simulink model "sim_SoftwareIntheLoop_Compensator"  (R2018a)
settings: Solver=ode3  StartTime=0.0  StopTime=40  FixedStep=0.005  RelTol=1e-3  EnableMultiTasking=on
InitFcn:
  | % load parameters of the default quadrotor
  | disp('Quadrotor parameters loaded by InitFcn')
  | parameters_estimationcontrol %load mdl_quadcopter as well!
  | 
  | % change to Simulation folder if in data folder
  | %cd([matlabpath '/Simulation']);
values from neighbouring files (symbols this model uses):
  controlHelperParams =     [LQR_param.mat]
  estimParams =     [LQR_param.mat]
  quad =     [LQR_param.mat]
  quadEDT =     [LQR_param.mat]
undefined symbols (not defined in the file or in its folder): DiscIntNeverNeededParam, Discrete, RSrun_sensordataCalib, rt_yout, Time
libraries: simulink x25, ctrlSharedLib x3
(part 1 of 2)
settings Model: Creator=ra  LastModifiedBy=Tony
settings DataIOCC: LimitDataPoints=on  SaveFormat=Array
settings OptimizationCC: LifeSpan=inf
settings DebuggingCC: SFUnexpectedBacktrackingDiag=warning  SFNoUnconditionalDefaultTransitionDiag=warning  SFExecutionAtInitializationDiag=none
settings HardwareCC: ProdBitPerPointer=32  ProdBitPerSizeT=32  ProdBitPerPtrDiffT=32  ProdLargestAtomicFloat=None  ProdIntDivRoundTo=Undefined  ProdEndianess=Unspecified  ProdWordSize=32  ProdHWDeviceType=32-bit Generic
settings ModelReferenceCC: PropagateSignalLabelsOutOfModel=off
settings CodeAppCC: StateflowObjectComments=on
settings GRTTargetCC: TargetLangStandard=C89/C90 (ANSI)  GeneratePreprocessorConditionals=Disable all
settings ConfigComp: CovMetricSettings=dw  CovHtmlReporting=on  CovSaveCumulativeToWorkspaceVar=on  CovSaveSingleToWorkspaceVar=on  CovExternalEMLEnable=off

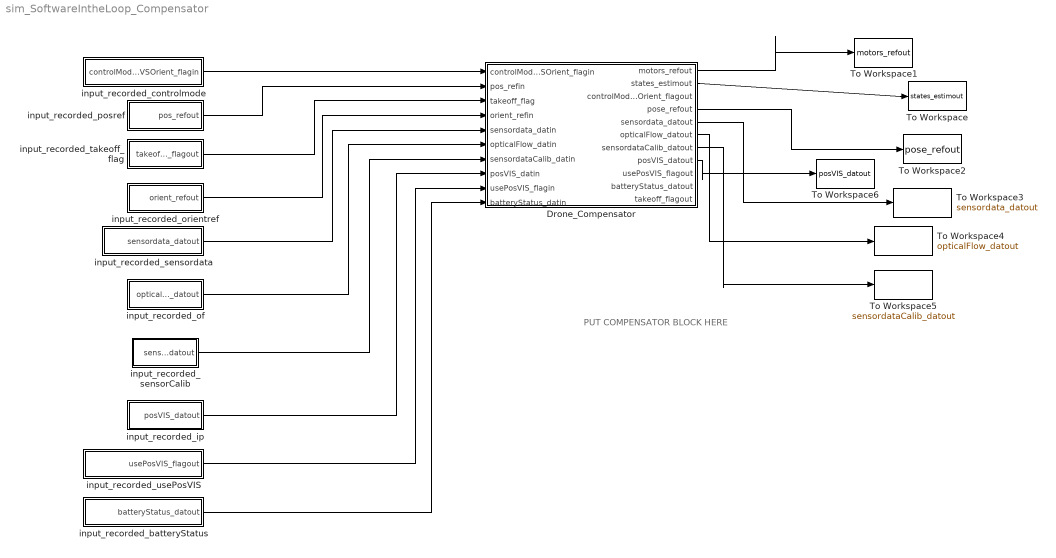
== system sim_SoftwareIntheLoop_Compensator ==
  note: PUT COMPENSATOR BLOCK HERE
  Drone_Compensator : Subsystem  TreatAsAtomicUnit=on
  To Workspace : ToWorkspace  VariableName=states_estimout  SaveFormat=Timeseries  SampleTime=-1
  To Workspace1 : ToWorkspace  VariableName=motors_refout  SaveFormat=Timeseries  SampleTime=-1
  To Workspace2 : ToWorkspace  VariableName=pose_refout  SaveFormat=Timeseries  SampleTime=-1
  To Workspace3 : ToWorkspace  VariableName=sensordata_datout  SaveFormat=Timeseries  SampleTime=-1
  To Workspace4 : ToWorkspace  VariableName=opticalFlow_datout  SaveFormat=Timeseries  SampleTime=-1
  To Workspace5 : ToWorkspace  VariableName=sensordataCalib_datout  SaveFormat=Timeseries  SampleTime=-1
  To Workspace6 : ToWorkspace  VariableName=posVIS_datout  SaveFormat=Timeseries  SampleTime=-1
  input_recorded_batteryStatus : Subsystem
  input_recorded_controlmode : Subsystem
  input_recorded_ip : Subsystem
  input_recorded_of : Subsystem
  input_recorded_orientref : Subsystem
  input_recorded_posref : Subsystem
  input_recorded_sensorCalib : Subsystem
  input_recorded_sensordata : Subsystem
  input_recorded_takeoff_flag : Subsystem
  input_recorded_usePosVIS : Subsystem
  wires:
  input_recorded_of/1(opticalFlow_datout) -> Drone_Compensator/6(opticalFlow_datin)
  input_recorded_sensordata/1(sensordata_datout) -> Drone_Compensator/5(sensordata_datin)
  input_recorded_ip/1(posVIS_datout) -> Drone_Compensator/8(posVIS_datin)
  input_recorded_orientref/1(orient_refout) -> Drone_Compensator/4(orient_refin)
  input_recorded_posref/1(pos_refout) -> Drone_Compensator/2(pos_refin)
  input_recorded_controlmode/1(controlModePosVSOrient_flagin) -> Drone_Compensator/1(controlModePosVSOrient_flagin)
  input_recorded_usePosVIS/1(usePosVIS_flagout) -> Drone_Compensator/9(usePosVIS_flagin)
  input_recorded_batteryStatus/1(batteryStatus_datout) -> Drone_Compensator/10(batteryStatus_datin)
  input_recorded_sensorCalib/1(sensordataCalib_datout) -> Drone_Compensator/7(sensordataCalib_datin)
  input_recorded_takeoff_flag/1(takeoff_flagout) -> Drone_Compensator/3(takeoff_flag)
  Drone_Compensator/2(states_estimout) -> To Workspace/1
  Drone_Compensator/1(motors_refout) -> To Workspace1/1
  Drone_Compensator/4(pose_refout) -> To Workspace2/1
  Drone_Compensator/5(sensordata_datout) -> To Workspace3/1
  Drone_Compensator/6(opticalFlow_datout) -> To Workspace4/1
  Drone_Compensator/7(sensordataCalib_datout) -> To Workspace5/1
  Drone_Compensator/8(posVIS_datout) -> To Workspace6/1

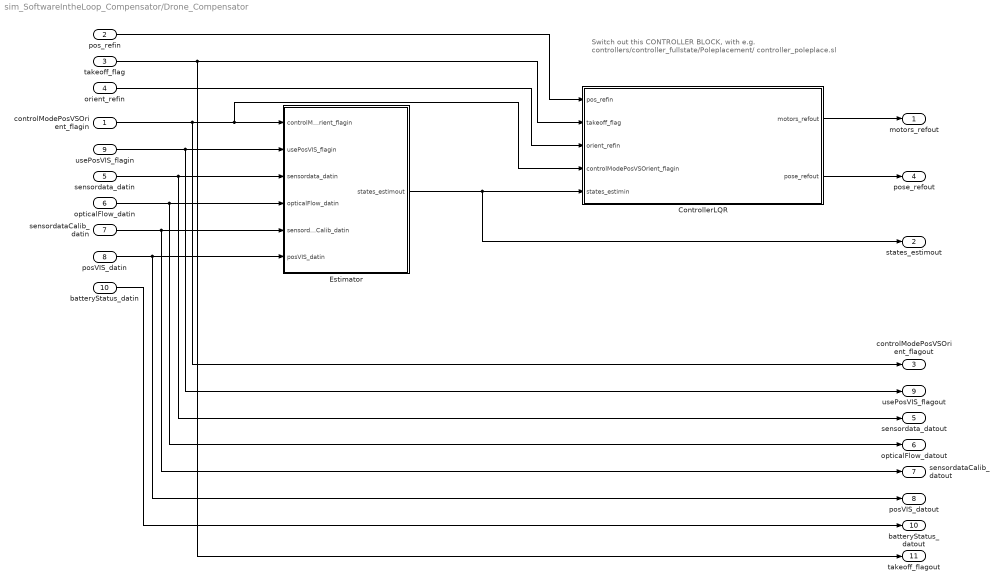
== system sim_SoftwareIntheLoop_Compensator/Drone_Compensator ==
  note: Switch out this CONTROLLER BLOCK, with e.g.
      | controllers/controller_fullstate/Poleplacement/
      | controller_poleplace.sl
  controlModePosVSOrient_flagin : Inport
  pos_refin : Inport  Port=2
  takeoff_flag : Inport  Port=3
  orient_refin : Inport  Port=4
  sensordata_datin : Inport  Port=5
  opticalFlow_datin : Inport  Port=6
  sensordataCalib_datin : Inport  Port=7
  posVIS_datin : Inport  Port=8
  usePosVIS_flagin : Inport  Port=9
  batteryStatus_datin : Inport  Port=10
  ControllerLQR : Subsystem  TreatAsAtomicUnit=on
  Estimator : Subsystem
  motors_refout : Outport
  states_estimout : Outport  Port=2
  controlModePosVSOrient_flagout : Outport  Port=3
  pose_refout : Outport  Port=4
  sensordata_datout : Outport  Port=5
  opticalFlow_datout : Outport  Port=6
  sensordataCalib_datout : Outport  Port=7
  posVIS_datout : Outport  Port=8
  usePosVIS_flagout : Outport  Port=9
  batteryStatus_datout : Outport  Port=10
  takeoff_flagout : Outport  Port=11
  wires:
  sensordata_datin/1 -> sensordata_datout/1, Estimator/3(sensordata_datin)
  pos_refin/1 -> ControllerLQR/1(pos_refin)
  Estimator/1(states_estimout) -> ControllerLQR/5(states_estimin), states_estimout/1
  orient_refin/1 -> ControllerLQR/3(orient_refin)
  controlModePosVSOrient_flagin/1 -> controlModePosVSOrient_flagout/1, ControllerLQR/4(controlModePosVSOrient_flagin), Estimator/1(controlModePosVSOrient_flagin)
  sensordataCalib_datin/1 -> sensordataCalib_datout/1, Estimator/5(sensordataCalib_datin)
  opticalFlow_datin/1 -> opticalFlow_datout/1, Estimator/4(opticalFlow_datin)
  posVIS_datin/1 -> posVIS_datout/1, Estimator/6(posVIS_datin)
  ControllerLQR/1(motors_refout) -> motors_refout/1
  usePosVIS_flagin/1 -> usePosVIS_flagout/1, Estimator/2(usePosVIS_flagin)
  ControllerLQR/2(pose_refout) -> pose_refout/1
  batteryStatus_datin/1 -> batteryStatus_datout/1
  takeoff_flag/1 -> ControllerLQR/2(takeoff_flag), takeoff_flagout/1

== system sim_SoftwareIntheLoop_Compensator/input_recorded_batteryStatus ==
  From Workspace : FromWorkspace  VariableName=RSrun_usePosVIS  SampleTime=quadEDT.sampletime
  Rate Transition : RateTransition  OutPortSampleTime=quadEDT.sampletime
  batteryStatus_datout : Outport
  wires:
  Rate Transition/1 -> batteryStatus_datout/1
  From Workspace/1 -> Rate Transition/1

== system sim_SoftwareIntheLoop_Compensator/input_recorded_controlmode ==
  From Workspace : FromWorkspace  VariableName=RSrun_controlMode  SampleTime=quadEDT.sampletime
  Rate Transition : RateTransition  OutPortSampleTime=quadEDT.sampletime
  controlModePosVSOrient_flagin : Outport
  wires:
  From Workspace/1 -> Rate Transition/1
  Rate Transition/1 -> controlModePosVSOrient_flagin/1

== system sim_SoftwareIntheLoop_Compensator/input_recorded_ip ==
  From Workspace : FromWorkspace  VariableName=RSrun_posVIS  SampleTime=quadEDT.sampletime
  Rate Transition : RateTransition  OutPortSampleTime=quadEDT.sampletime
  posVIS_datout : Outport
  wires:
  Rate Transition/1 -> posVIS_datout/1
  From Workspace/1 -> Rate Transition/1

== system sim_SoftwareIntheLoop_Compensator/input_recorded_of ==
  From Workspace : FromWorkspace  VariableName=RSrun_opticalFlow  SampleTime=quadEDT.sampletime
  Rate Transition : RateTransition  OutPortSampleTime=quadEDT.sampletime
  opticalFlow_datout : Outport
  wires:
  Rate Transition/1 -> opticalFlow_datout/1
  From Workspace/1 -> Rate Transition/1

== system sim_SoftwareIntheLoop_Compensator/input_recorded_orientref ==
  From Workspace : FromWorkspace  VariableName=RSrun_orient_ref  SampleTime=quadEDT.sampletime
  Rate Transition : RateTransition  OutPortSampleTime=quadEDT.sampletime
  orient_refout : Outport
  wires:
  From Workspace/1 -> Rate Transition/1
  Rate Transition/1 -> orient_refout/1

== system sim_SoftwareIntheLoop_Compensator/input_recorded_posref ==
  From Workspace : FromWorkspace  VariableName=RSrun_pos_ref  SampleTime=quadEDT.sampletime
  Rate Transition : RateTransition  OutPortSampleTime=quadEDT.sampletime
  pos_refout : Outport
  wires:
  Rate Transition/1 -> pos_refout/1
  From Workspace/1 -> Rate Transition/1

== system sim_SoftwareIntheLoop_Compensator/input_recorded_sensorCalib ==
  From Workspace : Constant  Value=RSrun_sensordataCalib  SampleTime=quadEDT.sampletime
  Rate Transition4 : RateTransition  OutPortSampleTime=quadEDT.sampletime
  sensorbias_default : Constant  Value=[0.09 -0.06 +0.337 -0.0095 -0.0075 0.0015 mean(rt_yout.signals(9).values(1:200))]  SampleTime=quadEDT.sampletime
  sensordataCalib_datout : Outport
  wires:
  From Workspace/1 -> Rate Transition4/1
  Rate Transition4/1 -> sensordataCalib_datout/1

== system sim_SoftwareIntheLoop_Compensator/input_recorded_sensordata ==
  Bus Creator : BusCreator  Inputs=8
  Demux : Demux  Outputs=8
  From Workspace : FromWorkspace  VariableName=RSrun_sensordata  SampleTime=quadEDT.sampletime
  Rate Transition : RateTransition  OutPortSampleTime=quadEDT.sampletime
  sensordata_datout : Outport
  wires:
  Demux/3 -> Bus Creator/3  "ddz"
  Demux/6 -> Bus Creator/6  "r"
  Demux/4 -> Bus Creator/4  "p"
  Demux/1 -> Bus Creator/1  "ddx"
  Demux/2 -> Bus Creator/2  "ddy"
  Bus Creator/1 -> Rate Transition/1
  Demux/5 -> Bus Creator/5  "q"
  From Workspace/1 -> Demux/1
  Demux/7 -> Bus Creator/7  "altitude_sonar"
  Rate Transition/1 -> sensordata_datout/1
  Demux/8 -> Bus Creator/8  "prs"

== system sim_SoftwareIntheLoop_Compensator/input_recorded_takeoff_flag ==
  From Workspace : FromWorkspace  VariableName=RSrun_takeoff_flag  SampleTime=quadEDT.sampletime
  Rate Transition : RateTransition  OutPortSampleTime=quadEDT.sampletime
  takeoff_flagout : Outport
  wires:
  Rate Transition/1 -> takeoff_flagout/1
  From Workspace/1 -> Rate Transition/1

== system sim_SoftwareIntheLoop_Compensator/input_recorded_usePosVIS ==
  From Workspace : FromWorkspace  VariableName=RSrun_usePosVIS  SampleTime=quadEDT.sampletime
  Rate Transition : RateTransition  OutPortSampleTime=quadEDT.sampletime
  usePosVIS_flagout : Outport
  wires:
  From Workspace/1 -> Rate Transition/1
  Rate Transition/1 -> usePosVIS_flagout/1

== system sim_SoftwareIntheLoop_Compensator/Drone_Compensator/ControllerLQR ==
  pos_refin : Inport
  takeoff_flag : Inport  Port=2
  orient_refin : Inport  Port=3
  controlModePosVSOrient_flagin : Inport  Port=4
  states_estimin : Inport  Port=5
  Add : Sum  Inputs=-+
  FullstateController : Subsystem
  Select pose : Selector  InputPortWidth=12  IndexOptions=Index vector (dialog)  Indices=[1:6]  OutputSizes=1
  SysteminputConverter : Subsystem
  statesReferences : Subsystem
  motors_refout : Outport
  pose_refout : Outport  Port=2
  wires:
  Select pose/1 -> pose_refout/1
  statesReferences/1(states_refout) -> Add/1, Select pose/1
  controlModePosVSOrient_flagin/1 -> statesReferences/3(controlModePosVSOrient_flagin)
  states_estimin/1 -> statesReferences/4(states_estimin), Add/2
  orient_refin/1 -> statesReferences/2(orient_refin)
  pos_refin/1 -> statesReferences/1(pos_refin)
  Add/1 -> FullstateController/1(state_error_datin)  "state error e"
  FullstateController/1(motors_refout) -> SysteminputConverter/2(motors_refin)
  SysteminputConverter/1(motors_refout) -> motors_refout/1
  takeoff_flag/1 -> SysteminputConverter/1(takeoffphase_flagin)

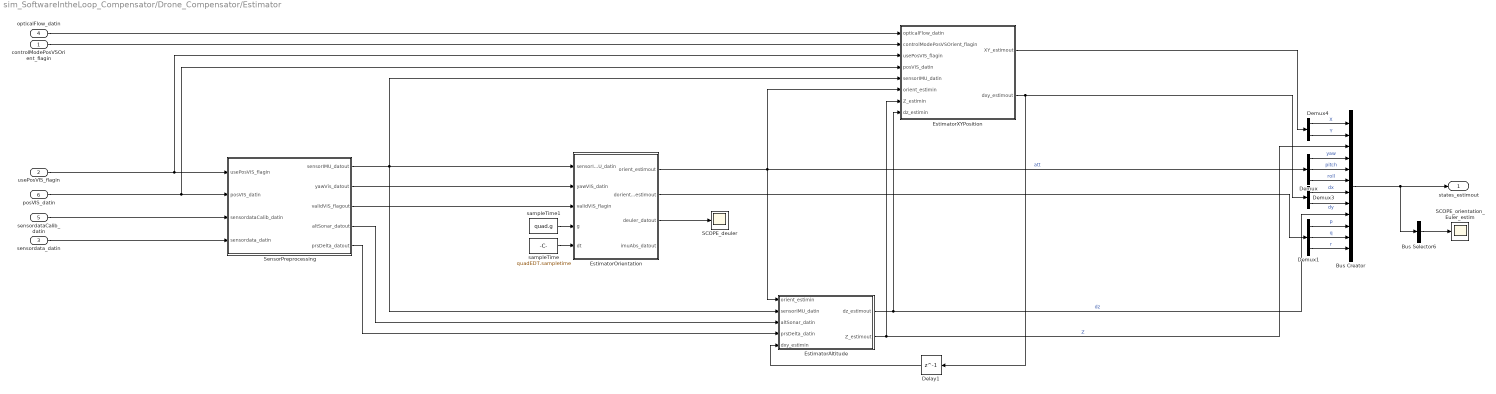
== system sim_SoftwareIntheLoop_Compensator/Drone_Compensator/Estimator ==
  controlModePosVSOrient_flagin : Inport
  usePosVIS_flagin : Inport  Port=2
  sensordata_datin : Inport  Port=3
  opticalFlow_datin : Inport  Port=4
  sensordataCalib_datin : Inport  Port=5
  posVIS_datin : Inport  Port=6
  Bus Creator : BusCreator  Inputs='X','Y','Z','yaw','pitch','roll','dx','dy','dz','p','q','r'
  Bus Selector6 : BusSelector  OutputSignals=yaw,pitch,roll  OutputAsBus=on
  Delay1 : Delay  DelayLength=1  InitialCondition=0
  Demux : Demux  Outputs=3
  Demux1 : Demux  Outputs=3
  Demux3 : Demux  Outputs=2
  Demux4 : Demux  Outputs=2
  EstimatorAltitude : Subsystem
  EstimatorOrientation : MATLAB Function  TreatAsAtomicUnit=on
  EstimatorXYPosition : Subsystem
  SCOPE_deuler : Scope
  SCOPE_orientation_Euler_estim : Scope
  SensorPreprocessing : Subsystem
  sampleTime : Constant  Value=quadEDT.sampletime  SampleTime=quadEDT.sampletime
  sampleTime1 : Constant  Value=quad.g  SampleTime=quadEDT.sampletime
  states_estimout : Outport
  wires:
  Bus Creator/1 -> Bus Selector6/1, states_estimout/1
  sampleTime/1 -> EstimatorOrientation/5(dt)
  sensordataCalib_datin/1 -> SensorPreprocessing/3(sensordataCalib_datin)
  EstimatorAltitude/2(Z_estimout) -> Bus Creator/3, EstimatorXYPosition/7(Z_estimin)  "Z"
  EstimatorAltitude/1(dz_estimout) -> EstimatorXYPosition/8(dz_estimin), Bus Creator/9  "dz"
  opticalFlow_datin/1 -> EstimatorXYPosition/1(opticalFlow_datin)
  Demux3/1 -> Bus Creator/7  "dx"
  Demux3/2 -> Bus Creator/8  "dy"
  EstimatorXYPosition/2(dxy_estimout) -> Delay1/1, Demux3/1
  Delay1/1 -> EstimatorAltitude/5(dxy_estimin)
  controlModePosVSOrient_flagin/1 -> EstimatorXYPosition/2(controlModePosVSOrient_flagin)
  Demux4/1 -> Bus Creator/1  "X"
  Demux4/2 -> Bus Creator/2  "Y"
  EstimatorXYPosition/1(XY_estimout) -> Demux4/1
  posVIS_datin/1 -> EstimatorXYPosition/4(posVIS_datin), SensorPreprocessing/2(posVIS_datin)
  usePosVIS_flagin/1 -> SensorPreprocessing/1(usePosVIS_flagin), EstimatorXYPosition/3(usePosVIS_flagin)
  Bus Selector6/1 -> SCOPE_orientation_Euler_estim/1
  SensorPreprocessing/1(sensorIMU_datout) -> EstimatorAltitude/2(sensorIMU_datin), EstimatorOrientation/1(sensorIMU_datin), EstimatorXYPosition/5(sensorIMU_datin)
  sensordata_datin/1 -> SensorPreprocessing/4(sensordata_datin)
  SensorPreprocessing/4(altSonar_datout) -> EstimatorAltitude/3(altSonar_datin)
  SensorPreprocessing/5(prsDelta_datout) -> EstimatorAltitude/4(prsDelta_datin)
  EstimatorOrientation/1(orient_estimout) -> EstimatorAltitude/1(orient_estimin), EstimatorXYPosition/6(orient_estimin), Demux/1  "att"
  Demux/2 -> Bus Creator/5  "pitch"
  Demux1/1 -> Bus Creator/10  "p"
  Demux1/2 -> Bus Creator/11  "q"
  Demux1/3 -> Bus Creator/12  "r"
  EstimatorOrientation/2(dorient_estimout) -> Demux1/1
  SensorPreprocessing/3(validVIS_flagout) -> EstimatorOrientation/3(validVIS_flagin)
  SensorPreprocessing/2(yawVis_datout) -> EstimatorOrientation/2(yawVIS_datin)
  Demux/3 -> Bus Creator/6  "roll"
  Demux/1 -> Bus Creator/4  "yaw"
  EstimatorOrientation/3(deuler_datout) -> SCOPE_deuler/1
  sampleTime1/1 -> EstimatorOrientation/4(g)

== system sim_SoftwareIntheLoop_Compensator/Drone_Compensator/ControllerLQR/FullstateController ==
  note: IMPLEMENT FULLSTATE-
      | CONTROLLER HERE
  state_error_datin : Inport
  "A " : Constant  Value=|  VectorParams1D=off
      | [0	0	0	0	0	0	1.00000000000000	0	0	0	0	0
      | 0	0	0	0	0	0	0	1.00000000000000	0	0	0	0
      | 0	0	0	0	0	0	0	0	1.00000000000000	0	0	0
      | 0	0	0	0	0	0	0	0	0	0	0	1.00000000000000
      | 0	0	0	0	0	0	0	0	0	0	1.00000000000000	0
      | 0	0	0	0	0	0	0	0	0	1.00000000000000	0	0
      | 0	0	0	0	-9.80999999983650	0	-0.0644051820480064	0	0	0	0.139009950032610	0
      | 0	0	0	0	0	9.80999999983650	3.94368000217969e-18	-0.0644051820480064	0	-0.139009950032610	-6.26098637146038e-20	-1.52055259660483e-19
      | 0	0	0	0	0	0	0	0	0	0	0	0
      | 0	0	0	0	0	0	0	-1.01355355109772	0	-2.18761944196916	0	0
      | 0	0	0	0	0	0	0.755758408753299	0	0	0	-1.63120319259874	0
      | 0	0	0	0	0	0	0	0	0	1.51387374186132e-16	0	-0.124838403164601]
  B : Constant  Value=|  VectorParams1D=off
      | [0	0	0	0
      | 0	0	0	0
      | 0	0	0	0
      | 0	0	0	0
      | 0	0	0	0
      | 0	0	0	0
      | 0	0	0	0
      | 0	0	0	0
      | -0.00960712392230772	0.00960712392230772	-0.00960712392230772	0.00960712392213385
      | 0.420192001834280	0.420192001834280	-0.420192001834280	-0.420192001834280
      | 0.313317079628604	-0.313317079628604	-0.313317079628604	0.313317079628604
      | -0.0115436310307942	-0.0115436310307942	-0.0115436310307942	-0.0115436310307942]
  Constant : Constant  Value=|  VectorParams1D=off
      | [-8.49718577324068	8.49718577324278	-25.4915573197690	-35.4049407217802	90.0682783196400	89.1568450104141	-11.6214164668536	11.5626871891982	-36.4857972458732	26.1882849112338	26.8528174312964	-44.1008245485000
      | 8.49718577324076	8.49718577324069	25.4915573196879	-35.4049407219011	-90.0682783196407	89.1568450104006	11.6214164668537	11.5626871892001	36.4857972458205	26.1882849112264	-26.8528174312965	-44.1008245487244
      | 8.49718577324275	-8.49718577324067	-25.4915573197688	-35.4049407217802	-90.0682783196551	-89.1568450104008	11.6214164668516	-11.5626871892001	-36.4857972458735	-26.1882849112264	-26.8528174313063	-44.1008245484999
      | -8.49718577324285	-8.49718577324278	25.4915573196756	-35.4049407219011	90.0682783196561	-89.1568450104140	-11.6214164668518	-11.5626871891982	36.4857972458054	-26.1882849112338	26.8528174313064	-44.1008245487245]
  K_lqr_toMotorcmd_slow : Constant  Value=|  VectorParams1D=off
      | [-11.3010583936794	11.3010583936810	-11.3010583936898	-47.0877433069619	118.606403302530	117.689229642168	-15.5706954566703	15.5112876366907	-24.4160285913130	34.5954570321764	35.2626383735406	-53.8321197902419
      | 11.3010583936794	11.3010583936790	11.3010583936727	-47.0877433070400	-118.606403302531	117.689229642160	15.5706954566704	15.5112876366922	24.4160285913003	34.5954570321714	-35.2626383735406	-53.8321197904123
      | 11.3010583936816	-11.3010583936788	-11.3010583936893	-47.0877433069617	-118.606403302539	-117.689229642159	15.5706954566690	-15.5112876366920	-24.4160285913129	-34.5954570321714	-35.2626383735473	-53.8321197902418
      | -11.3010583936815	-11.3010583936811	11.3010583936690	-47.0877433070397	118.606403302539	-117.689229642168	-15.5706954566690	-15.5112876366908	24.4160285912932	-34.5954570321764	35.2626383735473	-53.8321197904121]
  MATLAB Function : MATLAB Function  TreatAsAtomicUnit=on
  motors_refout : Outport
  wires:
  state_error_datin/1 -> MATLAB Function/2(x)
  MATLAB Function/1(u) -> motors_refout/1
  Constant/1 -> MATLAB Function/1(K)

== system sim_SoftwareIntheLoop_Compensator/Drone_Compensator/ControllerLQR/SysteminputConverter ==
  note: NOTE: The Systeminputconverter takes care of two things:
      | 1) During take off, adjust the total thrust proposed by the controller
      | 2) Translate the "mechanical" system inputs (total thrust, torques around body-frame x-y-z-axes) to actual motor commands.
      | This R4->R4 mapping is a simple bijective function and does not have any dynamics. This allows us to design the controller with more intuitive "mechanical inputs" (total thrust, torques) and later simple map these to actual motor commands.
  takeoffphase_flagin : Inport
  motors_refin : Inport  Port=2
  ControlMixer : Subsystem
  Conversion Motorcommands To TotalThrust and Torques : Subsystem
  Demux3 : Demux
  Takeoffphase_Thrustadjustment : Subsystem
  Thrust2Motorcmd : Subsystem
  motors_refout : Outport
  wires:
  takeoffphase_flagin/1 -> Takeoffphase_Thrustadjustment/1(takeoffphase_flagin)
  Takeoffphase_Thrustadjustment/1(totThrust_refout) -> ControlMixer/1(T_refin)
  Demux3/1 -> Takeoffphase_Thrustadjustment/2(totThrustbyController_refin)
  Demux3/4 -> ControlMixer/4(tau_roll)
  Demux3/3 -> ControlMixer/3(tau_pitch)
  Demux3/2 -> ControlMixer/2(tau_yaw)
  ControlMixer/1(thrusts_refout) -> Thrust2Motorcmd/1(thrusts_refin)
  Thrust2Motorcmd/1(motors_refout) -> motors_refout/1
  motors_refin/1 -> Conversion Motorcommands To TotalThrust and Torques/1(motors_refin)
  Conversion Motorcommands To TotalThrust and Torques/1(u_tthrust_torques) -> Demux3/1

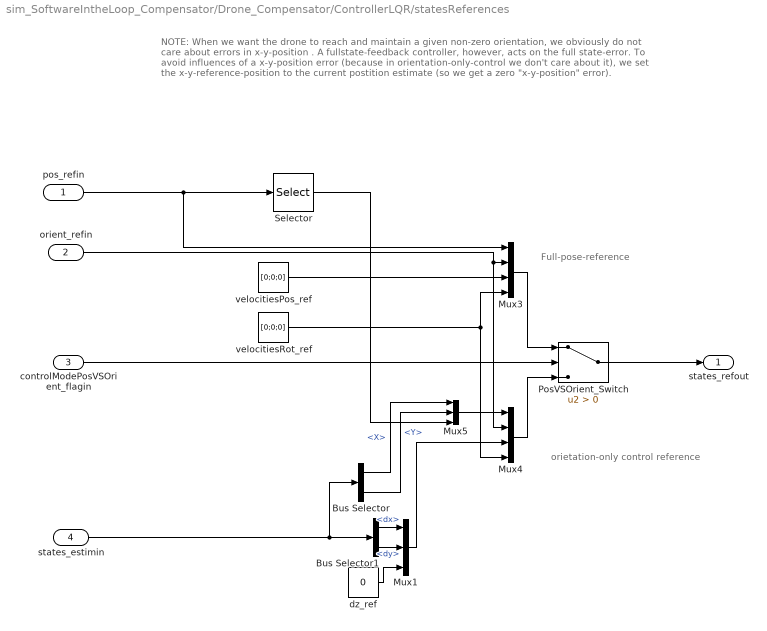
== system sim_SoftwareIntheLoop_Compensator/Drone_Compensator/ControllerLQR/statesReferences ==
  note: orietation-only control reference
  note: Full-pose-reference
  note: NOTE: When we want the drone to reach and maintain a given non-zero orientation,
      | we obviously do not care about errors in x-y-position . A fullstate-feedback controller, however, acts
      | on the full state-error. To avoid influences of a x-y-position error (because in orientation-only-control we don't care about it),
      | we set the x-y-reference-position to the current postition estimate (so we get a zero "x-y-position" error).
  pos_refin : Inport
  orient_refin : Inport  Port=2
  controlModePosVSOrient_flagin : Inport  Port=3
  states_estimin : Inport  Port=4
  Bus Selector : BusSelector  OutputSignals=X,Y
  Bus Selector1 : BusSelector  OutputSignals=dx,dy
  Mux1 : Mux  Inputs=3
  Mux3 : Mux
  Mux4 : Mux
  Mux5 : Mux  Inputs=3
  PosVSOrient_Switch : Switch  Criteria=u2 > Threshold
  Selector : Selector  InputPortWidth=3  IndexOptions=Index vector (dialog)  Indices=[3]  OutputSizes=1
  dz_ref : Constant  Value=0
  velocitiesPos_ref : Constant  Value=[0;0;0]
  velocitiesRot_ref : Constant  Value=[0;0;0]
  states_refout : Outport
  wires:
  dz_ref/1 -> Mux1/3
  Mux1/1 -> Mux4/3
  Bus Selector1/2 -> Mux1/2  "<dy>"
  Bus Selector1/1 -> Mux1/1  "<dx>"
  Mux5/1 -> Mux4/1
  Mux4/1 -> PosVSOrient_Switch/3
  Bus Selector/2 -> Mux5/2  "<Y>"
  Bus Selector/1 -> Mux5/1  "<X>"
  Mux3/1 -> PosVSOrient_Switch/1
  controlModePosVSOrient_flagin/1 -> PosVSOrient_Switch/2
  Selector/1 -> Mux5/3
  PosVSOrient_Switch/1 -> states_refout/1
  velocitiesRot_ref/1 -> Mux4/4, Mux3/4
  velocitiesPos_ref/1 -> Mux3/3
  states_estimin/1 -> Bus Selector/1, Bus Selector1/1
  orient_refin/1 -> Mux4/2, Mux3/2
  pos_refin/1 -> Mux3/1, Selector/1

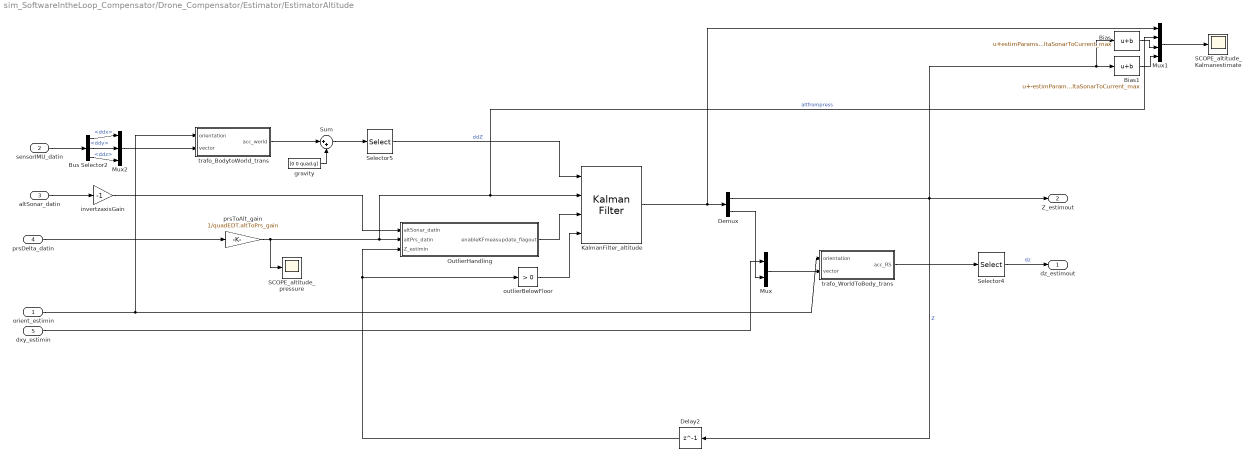
== system sim_SoftwareIntheLoop_Compensator/Drone_Compensator/Estimator/EstimatorAltitude ==
  orient_estimin : Inport
  sensorIMU_datin : Inport  Port=2
  altSonar_datin : Inport  Port=3
  prsDelta_datin : Inport  Port=4
  dxy_estimin : Inport  Port=5
  Bias : Bias  Bias=estimParams.alt.deltaSonarToCurrent_max
  Bias1 : Bias  Bias=-estimParams.alt.deltaSonarToCurrent_max
  Bus Selector2 : BusSelector  OutputSignals=ddx,ddy,ddz
  Delay2 : Delay  DelayLength=1  InitialCondition=0
  Demux : Demux  Outputs=2
  KalmanFilter_altitude : ctrlSharedLib/Kalman Filter  TimeDomain=Discrete-Time  UseCurrentEstimator=on  ModelSource=Individual A, B, C, D matrices  ModelSourceVariable=sys  A=[1 quadEDT.sampletime; 0 1]  B=[0;quadEDT.sampletime]  C=[1 0]  D=[0]  NumberOfStates=2  NumberOfInputs=2  NumberOfOutputs=2  InitialEstimateSource=Dialog  X0=[-0.046 0]  P0=10  UseK=off  UseGH=on  NumberOfProcessNoiseInputs=2  G=estimParams.alt.kf.G  TimeInvariantG=on  H=estimParams.alt.kf.H  TimeInvariantH=on  Q=0.0478  TimeInvariantQ=on  R=0.0082  TimeInvariantR=on  N=estimParams.alt.kf.N  TimeInvariantN=on  AddInputPort=on  AddEnablePort=on  ExternalReset=Level hold  OutputEstimatedY=off  OutputP=off  Ts=-1
      settings: SourceProductBaseCode=CT
  Mux : Mux  Inputs=2
  Mux1 : Mux
  Mux2 : Mux  Inputs=3
  OutlierHandling : Subsystem
  SCOPE_altitude_Kalmanestimate : Scope
  SCOPE_altitude_pressure : Scope
  Selector4 : Selector  InputPortWidth=3  IndexOptions=Index vector (dialog)  Indices=[3]  OutputSizes=1
  Selector5 : Selector  InputPortWidth=3  IndexOptions=Index vector (dialog)  Indices=[3]  OutputSizes=1
  Sum : Sum  Inputs=|++
  gravity : Constant  Value=[0 0 quad.g]
  invertzaxisGain : Gain  Gain=-1
  outlierBelowFloor : simulink/Logic and Bit Operations/Compare To Constant  relop=>  const=0  OutDataTypeStr=boolean
  prsToAlt_gain : Gain  Gain=1/quadEDT.altToPrs_gain
  trafo_BodytoWorld_trans : MATLAB Function  TreatAsAtomicUnit=on
  trafo_WorldToBody_trans : MATLAB Function  TreatAsAtomicUnit=on
  dz_estimout : Outport
  Z_estimout : Outport  Port=2
  wires:
  orient_estimin/1 -> trafo_BodytoWorld_trans/1(orientation), trafo_WorldToBody_trans/1(orientation)
  altSonar_datin/1 -> invertzaxisGain/1
  trafo_BodytoWorld_trans/1(acc_world) -> Sum/1
  gravity/1 -> Sum/2
  Sum/1 -> Selector5/1
  KalmanFilter_altitude/1 -> Mux1/1, Demux/1
  Mux/1 -> trafo_WorldToBody_trans/2(vector)
  Selector5/1 -> KalmanFilter_altitude/1  "ddZ"
  invertzaxisGain/1 -> OutlierHandling/1(altSonar_datin)
  Demux/1 -> Bias1/1, Bias/1, Delay2/1, Z_estimout/1  "Z"
  Selector4/1 -> dz_estimout/1  "dz"
  Demux/2 -> Mux/2
  Mux1/1 -> SCOPE_altitude_Kalmanestimate/1
  Bias/1 -> Mux1/3
  Bias1/1 -> Mux1/4
  outlierBelowFloor/1 -> KalmanFilter_altitude/4
  prsDelta_datin/1 -> prsToAlt_gain/1
  prsToAlt_gain/1 -> SCOPE_altitude_pressure/1, Mux1/2, KalmanFilter_altitude/2, OutlierHandling/2(altPrs_datin)  "altfrompress"
  Delay2/1 -> outlierBelowFloor/1, OutlierHandling/3(Z_estimin)
  OutlierHandling/1(enableKFmeasupdate_flagout) -> KalmanFilter_altitude/3
  dxy_estimin/1 -> Mux/1
  trafo_WorldToBody_trans/1(acc_RS) -> Selector4/1
  Bus Selector2/1 -> Mux2/1  "<ddx>"
  Bus Selector2/2 -> Mux2/2  "<ddy>"
  Bus Selector2/3 -> Mux2/3  "<ddz>"
  sensorIMU_datin/1 -> Bus Selector2/1
  Mux2/1 -> trafo_BodytoWorld_trans/2(vector)

== system sim_SoftwareIntheLoop_Compensator/Drone_Compensator/Estimator/EstimatorXYPosition ==
  opticalFlow_datin : Inport
  controlModePosVSOrient_flagin : Inport  Port=2
  usePosVIS_flagin : Inport  Port=3
  posVIS_datin : Inport  Port=4
  sensorIMU_datin : Inport  Port=5
  orient_estimin : Inport  Port=6
  Z_estimin : Inport  Port=7
  dz_estimin : Inport  Port=8
  EstimatorVelocity : Subsystem
  EstimatorXYPosition : Subsystem
  XY_estimout : Outport
  dxy_estimout : Outport  Port=2
  wires:
  orient_estimin/1 -> EstimatorVelocity/4(orient_estimin), EstimatorXYPosition/2(orient_estimin)
  EstimatorVelocity/1(dxy_estimout) -> EstimatorXYPosition/1(dxy_estimin), dxy_estimout/1
  opticalFlow_datin/1 -> EstimatorVelocity/1(opticalFlow_datin)
  sensorIMU_datin/1 -> EstimatorVelocity/3(sensorIMU_datin)
  Z_estimin/1 -> EstimatorVelocity/2(Z_estimin)
  controlModePosVSOrient_flagin/1 -> EstimatorXYPosition/3(controlModePosVSOrient_flagin)
  dz_estimin/1 -> EstimatorXYPosition/4(dz_estimin)
  posVIS_datin/1 -> EstimatorXYPosition/5(posVIS_datin)
  usePosVIS_flagin/1 -> EstimatorXYPosition/6(usePosVIS_flagin)
  EstimatorXYPosition/1(XY_estimout) -> XY_estimout/1

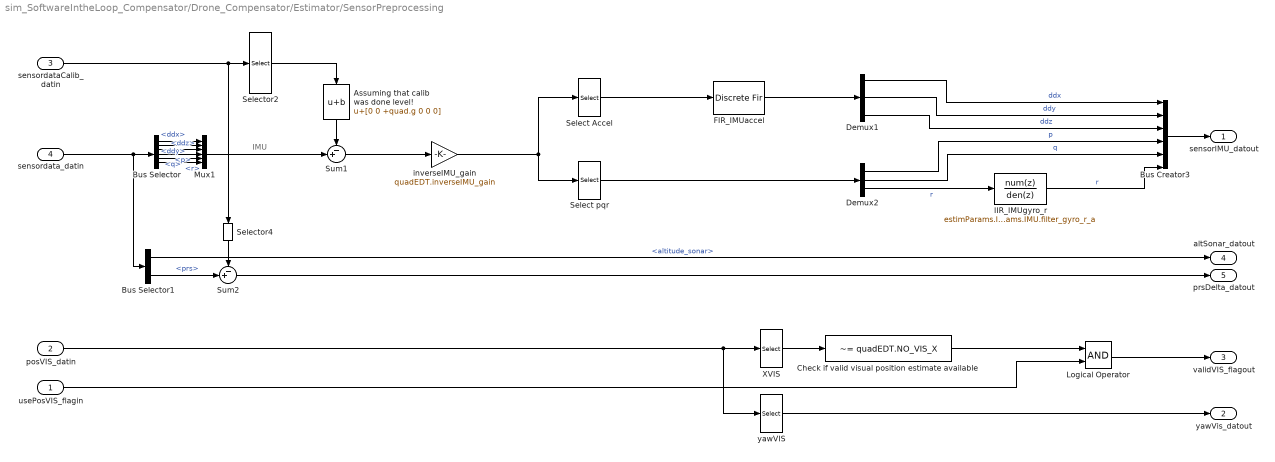
== system sim_SoftwareIntheLoop_Compensator/Drone_Compensator/Estimator/SensorPreprocessing ==
  note: IMU
  usePosVIS_flagin : Inport
  posVIS_datin : Inport  Port=2
  sensordataCalib_datin : Inport  Port=3
  sensordata_datin : Inport  Port=4
  Assuming that calib was done level! : Bias  Bias=[0 0 +quad.g 0 0 0]
  Bus Creator3 : BusCreator  Inputs=6
  Bus Selector : BusSelector  OutputSignals=ddx,ddy,ddz,p,q,r
  Bus Selector1 : BusSelector  OutputSignals=altitude_sonar,prs
  Check if valid visual position estimate available : simulink/Logic and Bit Operations/Compare To Constant  relop=~=  const=quadEDT.NO_VIS_X  OutDataTypeStr=boolean
  Demux1 : Demux  Outputs=3
  Demux2 : Demux  Outputs=3
  FIR_IMUaccel : DiscreteFir  Coefficients=estimParams.IMU.filter_accel.Coefficients
  IIR_IMUgyro_r : DiscreteFilter  Numerator=estimParams.IMU.filter_gyro_r_b  Denominator=estimParams.IMU.filter_gyro_r_a
  Logical Operator : Logic  AllPortsSameDT=off  OutDataTypeStr=boolean
  Mux1 : Mux  Inputs=6
  Select Accel : Selector  InputPortWidth=6  IndexOptions=Index vector (dialog)  Indices=[1 2 3]  OutputSizes=1
  Select pqr : Selector  InputPortWidth=6  IndexOptions=Index vector (dialog)  Indices=[4 5 6]  OutputSizes=1
  Selector2 : Selector  InputPortWidth=7  IndexOptions=Index vector (dialog)  Indices=[1:6]  OutputSizes=1
  Selector4 : Selector  InputPortWidth=7  IndexOptions=Index vector (dialog)  Indices=[7]  OutputSizes=1
  Sum1 : Sum  Inputs=-+|
  Sum2 : Sum  Inputs=-+|
  XVIS : Selector  InputPortWidth=4  IndexOptions=Index vector (dialog)  Indices=1  OutputSizes=1
  inverseIMU_gain : Gain  Gain=quadEDT.inverseIMU_gain
  yawVIS : Selector  InputPortWidth=4  IndexOptions=Index vector (dialog)  Indices=4  OutputSizes=1
  sensorIMU_datout : Outport
  yawVis_datout : Outport  Port=2
  validVIS_flagout : Outport  Port=3
  altSonar_datout : Outport  Port=4
  prsDelta_datout : Outport  Port=5
  wires:
  posVIS_datin/1 -> yawVIS/1, XVIS/1
  Bus Creator3/1 -> sensorIMU_datout/1
  Demux1/1 -> Bus Creator3/1  "ddx"
  Demux1/2 -> Bus Creator3/2  "ddy"
  Demux1/3 -> Bus Creator3/3  "ddz"
  Sum1/1 -> inverseIMU_gain/1
  Selector2/1 -> Assuming that calib was done level!/1
  Demux2/1 -> Bus Creator3/4  "p"
  Demux2/2 -> Bus Creator3/5  "q"
  inverseIMU_gain/1 -> Select pqr/1, Select Accel/1
  Select Accel/1 -> FIR_IMUaccel/1
  FIR_IMUaccel/1 -> Demux1/1
  Demux2/3 -> IIR_IMUgyro_r/1  "r"
  IIR_IMUgyro_r/1 -> Bus Creator3/6  "r"
  sensordataCalib_datin/1 -> Selector4/1, Selector2/1
  Bus Selector/1 -> Mux1/1  "<ddx>"
  Bus Selector/2 -> Mux1/2  "<ddy>"
  Bus Selector/3 -> Mux1/3  "<ddz>"
  Bus Selector/4 -> Mux1/4  "<p>"
  Bus Selector/5 -> Mux1/5  "<q>"
  Bus Selector/6 -> Mux1/6  "<r>"
  sensordata_datin/1 -> Bus Selector1/1, Bus Selector/1
  Bus Selector1/1 -> altSonar_datout/1  "<altitude_sonar>"
  Selector4/1 -> Sum2/1
  Bus Selector1/2 -> Sum2/2  "<prs>"
  Sum2/1 -> prsDelta_datout/1
  Mux1/1 -> Sum1/2
  XVIS/1 -> Check if valid visual position estimate available/1
  yawVIS/1 -> yawVis_datout/1
  Logical Operator/1 -> validVIS_flagout/1
  Check if valid visual position estimate available/1 -> Logical Operator/1
  usePosVIS_flagin/1 -> Logical Operator/2
  Assuming that calib was done level!/1 -> Sum1/1
  Select pqr/1 -> Demux2/1

== system sim_SoftwareIntheLoop_Compensator/Drone_Compensator/ControllerLQR/SysteminputConverter/ControlMixer ==
  note: NOTE: The controlmixer translates total thrust and the three torque inputs that the controller came up with into 'thrust per motor'.
  T_refin : Inport
  tau_yaw : Inport  Port=2
  tau_pitch : Inport  Port=3
  tau_roll : Inport  Port=4
  Mux2 : Mux
  Product : Product  Multiplication=Matrix(*)  RndMeth=Zero
  Saturation2 : Saturate  UpperLimit=-0.05*controlHelperParams.motorsThrustperMotor_max  LowerLimit=-controlHelperParams.motorsThrustperMotor_max
  TorquetotalThrustToThrustperMotor : Constant  Value=controlHelperParams.Q2Ts
  thrusts_refout : Outport
  wires:
  tau_roll/1 -> Mux2/4
  tau_pitch/1 -> Mux2/3
  tau_yaw/1 -> Mux2/2
  T_refin/1 -> Mux2/1
  Product/1 -> Saturation2/1
  TorquetotalThrustToThrustperMotor/1 -> Product/1
  Mux2/1 -> Product/2
  Saturation2/1 -> thrusts_refout/1

== system sim_SoftwareIntheLoop_Compensator/Drone_Compensator/ControllerLQR/SysteminputConverter/Conversion Motorcommands To TotalThrust and Torques ==
  motors_refin : Inport
  MotorsRotationDirection : Gain  Gain=diag([-1,1,-1,1])  Multiplication=Matrix(K*u)
  ThrustperMotor To TotalThrust and Torques : Gain  Gain=controlHelperParams.Ts2Q  Multiplication=Matrix(K*u)
  W2ToThrust : Gain  Gain=quadEDT.w2ToThrust_gain
  motorsToW2_Gain : Gain  Gain=quadEDT.motorcommandToW2_gain
  u_tthrust_torques : Outport
  wires:
  ThrustperMotor To TotalThrust and Torques/1 -> u_tthrust_torques/1
  motors_refin/1 -> MotorsRotationDirection/1
  W2ToThrust/1 -> ThrustperMotor To TotalThrust and Torques/1
  motorsToW2_Gain/1 -> W2ToThrust/1
  MotorsRotationDirection/1 -> motorsToW2_Gain/1

== system sim_SoftwareIntheLoop_Compensator/Drone_Compensator/ControllerLQR/SysteminputConverter/Takeoffphase_Thrustadjustment ==
  note: NOTE: Below 40cm in altitude, sonar measurements and camera data are very unreliable.
      | We therefore introduce a take-off phase where the drone controls attitude only and runs an uncontrolled total thrust of takeofff_Gain/100  % above equilibrium thrust.
  takeoffphase_flagin : Inport
  totThrustbyController_refin : Inport  Port=2
  Add1 : Sum  Inputs=++|
  HoverThrustLinearizationPoint : Constant  Value=-quad.g*quad.M
  "SCOPE_totalthrust " : Scope
  SaturationThrust : Saturate  UpperLimit=controlHelperParams.totalThrust_maxRelative*controlHelperParams.motorsThrustperMotor_max*4  LowerLimit=-controlHelperParams.totalThrust_maxRelative*controlHelperParams.motorsThrustperMotor_max*4
  TakeoffOrControl_Switch : Switch  Criteria=u2 > Threshold
  takeoff_gain : Gain  Gain=controlHelperParams.takeoff_gain
  totThrust_refout : Outport
  wires:
  takeoffphase_flagin/1 -> TakeoffOrControl_Switch/2
  SaturationThrust/1 -> totThrust_refout/1, "SCOPE_totalthrust "/1
  TakeoffOrControl_Switch/1 -> Add1/2
  takeoff_gain/1 -> TakeoffOrControl_Switch/1
  HoverThrustLinearizationPoint/1 -> Add1/1, takeoff_gain/1
  totThrustbyController_refin/1 -> TakeoffOrControl_Switch/3
  Add1/1 -> SaturationThrust/1

== system sim_SoftwareIntheLoop_Compensator/Drone_Compensator/ControllerLQR/SysteminputConverter/Thrust2Motorcmd ==
  note: NOTE: This block translates thrust per motor into a command that is acutally send to the motors.
  thrusts_refin : Inport
  MotorsRotationDirection : Gain  Gain=[-1,1,-1,1]
  Signed Sqrt : Sqrt  Operator=signedSqrt  SaturateOnIntegerOverflow=on
  ThrustToW2_Gain : Gain  Gain=1/quadEDT.w2ToThrust_gain
  W2ToMotorsCmd_Gain : Gain  Gain=1/quadEDT.motorcommandToW2_gain
  motors_refout : Outport
  wires:
  MotorsRotationDirection/1 -> W2ToMotorsCmd_Gain/1, Signed Sqrt/1
  Signed Sqrt/1 -> ?  "w"
  W2ToMotorsCmd_Gain/1 -> motors_refout/1
  thrusts_refin/1 -> ThrustToW2_Gain/1
  ThrustToW2_Gain/1 -> MotorsRotationDirection/1

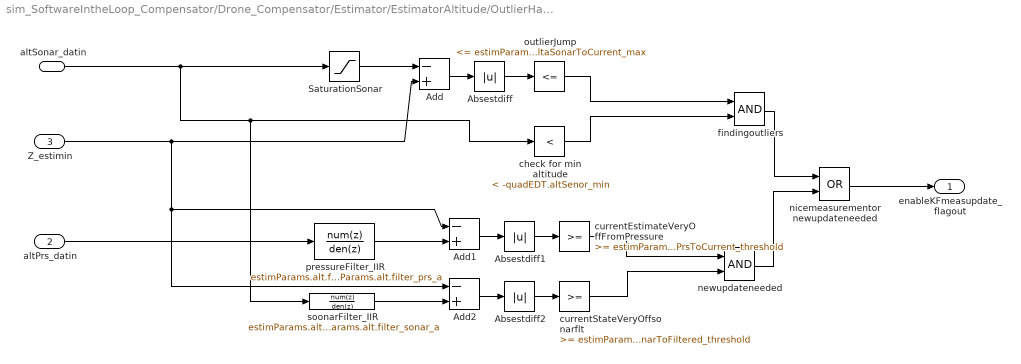
== system sim_SoftwareIntheLoop_Compensator/Drone_Compensator/Estimator/EstimatorAltitude/OutlierHandling ==
  altSonar_datin : Inport
  altPrs_datin : Inport  Port=2
  Z_estimin : Inport  Port=3
  Absestdiff : Abs
  Absestdiff1 : Abs
  Absestdiff2 : Abs
  Add : Sum  Inputs=-+
  Add1 : Sum  Inputs=-+
  Add2 : Sum  Inputs=-+
  SaturationSonar : Saturate  UpperLimit=-quadEDT.altSenor_min  LowerLimit=-inf
  check for min altitude : simulink/Logic and Bit Operations/Compare To Constant  relop=<  const=-quadEDT.altSenor_min  OutDataTypeStr=boolean
  currentEstimateVeryOffFromPressure : simulink/Logic and Bit Operations/Compare To Constant  relop=>=  const=estimParams.alt.deltaPrsToCurrent_threshold  OutDataTypeStr=boolean
  currentStateVeryOffsonarflt : simulink/Logic and Bit Operations/Compare To Constant  relop=>=  const=estimParams.alt.deltaSonarToFiltered_threshold  OutDataTypeStr=boolean
  findingoutliers : Logic  AllPortsSameDT=off  OutDataTypeStr=boolean
  newupdateneeded : Logic  AllPortsSameDT=off  OutDataTypeStr=boolean
  nicemeasurementor newupdateneeded : Logic  Operator=OR  AllPortsSameDT=off  OutDataTypeStr=boolean
  outlierJump : simulink/Logic and Bit Operations/Compare To Constant  relop=<=  const=estimParams.alt.deltaSonarToCurrent_max  OutDataTypeStr=boolean
  pressureFilter_IIR : DiscreteFilter  Numerator=estimParams.alt.filter_prs_b  Denominator=estimParams.alt.filter_prs_a
  soonarFilter_IIR : DiscreteFilter  Numerator=estimParams.alt.filter_sonar_b  Denominator=estimParams.alt.filter_sonar_a
  enableKFmeasupdate_flagout : Outport
  wires:
  Absestdiff1/1 -> currentEstimateVeryOffFromPressure/1
  soonarFilter_IIR/1 -> Add2/2
  altPrs_datin/1 -> pressureFilter_IIR/1
  pressureFilter_IIR/1 -> Add1/2
  currentStateVeryOffsonarflt/1 -> newupdateneeded/2
  Add2/1 -> Absestdiff2/1
  Z_estimin/1 -> Add/2, Add2/1, Add1/1
  currentEstimateVeryOffFromPressure/1 -> newupdateneeded/1
  altSonar_datin/1 -> soonarFilter_IIR/1, check for min altitude/1, SaturationSonar/1
  Absestdiff2/1 -> currentStateVeryOffsonarflt/1
  newupdateneeded/1 -> nicemeasurementor newupdateneeded/2
  Add/1 -> Absestdiff/1
  Absestdiff/1 -> outlierJump/1
  SaturationSonar/1 -> Add/1
  outlierJump/1 -> findingoutliers/1
  check for min altitude/1 -> findingoutliers/2
  findingoutliers/1 -> nicemeasurementor newupdateneeded/1
  nicemeasurementor newupdateneeded/1 -> enableKFmeasupdate_flagout/1
  Add1/1 -> Absestdiff1/1

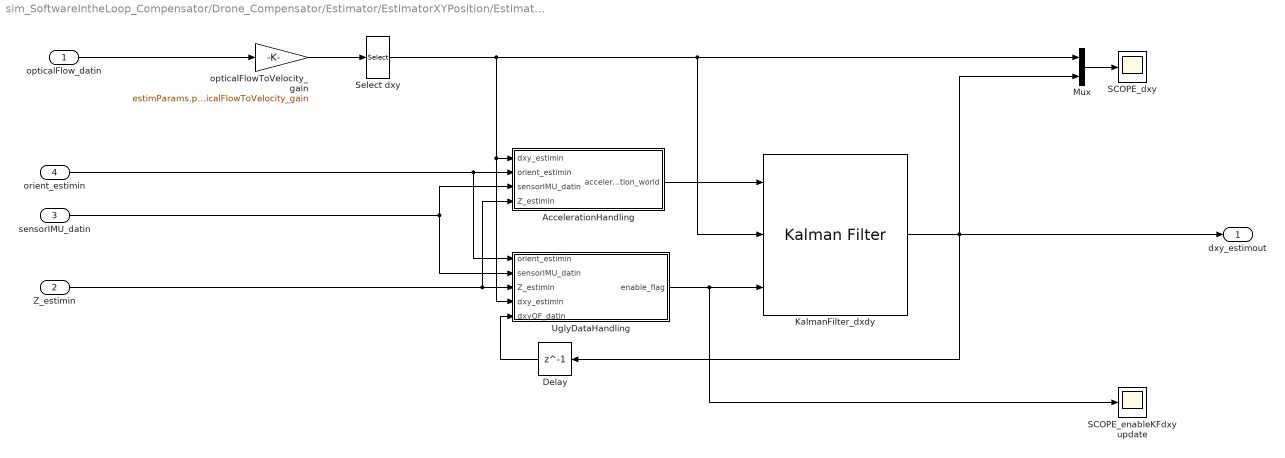
== system sim_SoftwareIntheLoop_Compensator/Drone_Compensator/Estimator/EstimatorXYPosition/EstimatorVelocity ==
  opticalFlow_datin : Inport
  Z_estimin : Inport  Port=2
  sensorIMU_datin : Inport  Port=3
  orient_estimin : Inport  Port=4
  AccelerationHandling : Subsystem
  Delay : Delay  DelayLength=1  InitialCondition=0
  KalmanFilter_dxdy : ctrlSharedLib/Kalman Filter  TimeDomain=Discrete-Time  UseCurrentEstimator=on  ModelSource=Individual A, B, C, D matrices  ModelSourceVariable=ss(0.95,1,1,0,1)  A=eye(2)  B=quadEDT.sampletime*eye(2)  C=eye(2)  D=0  NumberOfStates=1  NumberOfInputs=1  NumberOfOutputs=1  InitialEstimateSource=Dialog  X0=0  P0=10  UseK=off  UseGH=on  NumberOfProcessNoiseInputs=1  G=estimParams.pos.kfvelo.G  TimeInvariantG=on  H=estimParams.pos.kfvelo.H  TimeInvariantH=on  Q=estimParams.pos.kfvelo.Q  TimeInvariantQ=on  R=estimParams.pos.kfvelo.R  TimeInvariantR=on  N=estimParams.pos.kfvelo.N  TimeInvariantN=on  AddInputPort=on  AddEnablePort=on  OutputEstimatedY=off  OutputP=off  Ts=-1
      settings: SourceProductBaseCode=CT
  Mux : Mux  Inputs=2
  SCOPE_dxy : Scope
  SCOPE_enableKFdxyupdate : Scope
  Select dxy : Selector  InputPortWidth=3  IndexOptions=Index vector (dialog)  Indices=[1 2]  OutputSizes=1
  UglyDataHandling : Subsystem
  opticalFlowToVelocity_gain : Gain  Gain=estimParams.pos.opticalFlowToVelocity_gain
  dxy_estimout : Outport
  wires:
  orient_estimin/1 -> AccelerationHandling/2(orient_estimin), UglyDataHandling/1(orient_estimin)
  sensorIMU_datin/1 -> AccelerationHandling/3(sensorIMU_datin), UglyDataHandling/2(sensorIMU_datin)
  opticalFlow_datin/1 -> opticalFlowToVelocity_gain/1
  Select dxy/1 -> AccelerationHandling/1(dxy_estimin), UglyDataHandling/4(dxy_estimin), KalmanFilter_dxdy/2, Mux/1
  opticalFlowToVelocity_gain/1 -> Select dxy/1
  KalmanFilter_dxdy/1 -> Mux/2, dxy_estimout/1, Delay/1
  UglyDataHandling/1(enable_flag) -> SCOPE_enableKFdxyupdate/1, KalmanFilter_dxdy/3
  Z_estimin/1 -> AccelerationHandling/4(Z_estimin), UglyDataHandling/3(Z_estimin)
  Mux/1 -> SCOPE_dxy/1
  AccelerationHandling/1(acceleration_world) -> KalmanFilter_dxdy/1
  Delay/1 -> UglyDataHandling/5(dxyOF_datin)

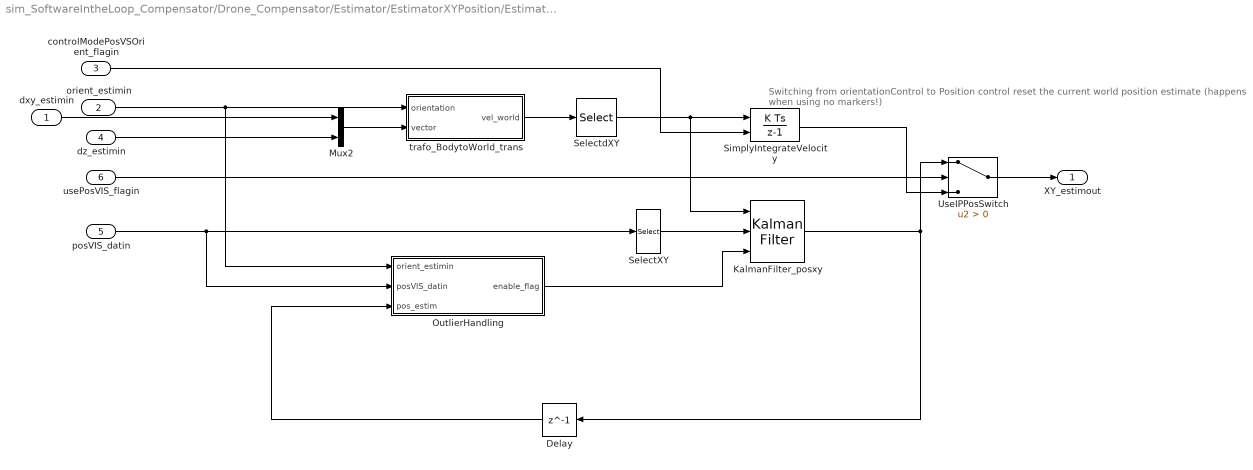
== system sim_SoftwareIntheLoop_Compensator/Drone_Compensator/Estimator/EstimatorXYPosition/EstimatorXYPosition ==
  note: Switching from orientationControl to Position control reset the current world position estimate (happens when using no markers!)
  dxy_estimin : Inport
  orient_estimin : Inport  Port=2
  controlModePosVSOrient_flagin : Inport  Port=3
  dz_estimin : Inport  Port=4
  posVIS_datin : Inport  Port=5
  usePosVIS_flagin : Inport  Port=6
  Delay : Delay  DelayLength=1  InitialCondition=0
  KalmanFilter_posxy : ctrlSharedLib/Kalman Filter  TimeDomain=Discrete-Time  UseCurrentEstimator=on  ModelSource=Individual A, B, C, D matrices  ModelSourceVariable=ss(0.95,1,1,0,1)  A=eye(2)  B=quadEDT.sampletime*eye(2)  C=eye(2)  D=0  NumberOfStates=1  NumberOfInputs=1  NumberOfOutputs=1  InitialEstimateSource=Dialog  X0=[.1 0.0]  P0=10  UseK=off  UseGH=on  NumberOfProcessNoiseInputs=1  G=estimParams.pos.kfpos.G  TimeInvariantG=on  H=estimParams.pos.kfpos.H  TimeInvariantH=on  Q=estimParams.pos.kfpos.Q  TimeInvariantQ=on  R=estimParams.pos.kfpos.R  TimeInvariantR=on  N=estimParams.pos.kfpos.N  TimeInvariantN=on  AddInputPort=on  AddEnablePort=on  OutputEstimatedY=off  OutputP=off  Ts=-1
      settings: SourceProductBaseCode=CT
  Mux2 : Mux  Inputs=2
  OutlierHandling : Subsystem
  SelectXY : Selector  InputPortWidth=4  IndexOptions=Index vector (dialog)  Indices=[1 2]  OutputSizes=1
  SelectdXY : Selector  InputPortWidth=3  IndexOptions=Index vector (dialog)  Indices=[1 2]  OutputSizes=1
  SimplyIntegrateVelocity : DiscreteIntegrator  ExternalReset=rising  SampleTime=quadEDT.sampletime  ICPrevOutput=DiscIntNeverNeededParam  ICPrevScaledInput=DiscIntNeverNeededParam
  UseIPPosSwitch : Switch  Criteria=u2 > Threshold
  trafo_BodytoWorld_trans : MATLAB Function  TreatAsAtomicUnit=on
  XY_estimout : Outport
  wires:
  orient_estimin/1 -> trafo_BodytoWorld_trans/1(orientation), OutlierHandling/1(orient_estimin)
  dxy_estimin/1 -> Mux2/1
  SimplyIntegrateVelocity/1 -> UseIPPosSwitch/3
  dz_estimin/1 -> Mux2/2
  Mux2/1 -> trafo_BodytoWorld_trans/2(vector)
  trafo_BodytoWorld_trans/1(vel_world) -> SelectdXY/1
  SelectdXY/1 -> KalmanFilter_posxy/1, SimplyIntegrateVelocity/1
  posVIS_datin/1 -> SelectXY/1, OutlierHandling/2(posVIS_datin)
  KalmanFilter_posxy/1 -> Delay/1, UseIPPosSwitch/1
  controlModePosVSOrient_flagin/1 -> SimplyIntegrateVelocity/2
  UseIPPosSwitch/1 -> XY_estimout/1
  usePosVIS_flagin/1 -> UseIPPosSwitch/2
  SelectXY/1 -> KalmanFilter_posxy/2
  OutlierHandling/1(enable_flag) -> KalmanFilter_posxy/3
  Delay/1 -> OutlierHandling/3(pos_estim)

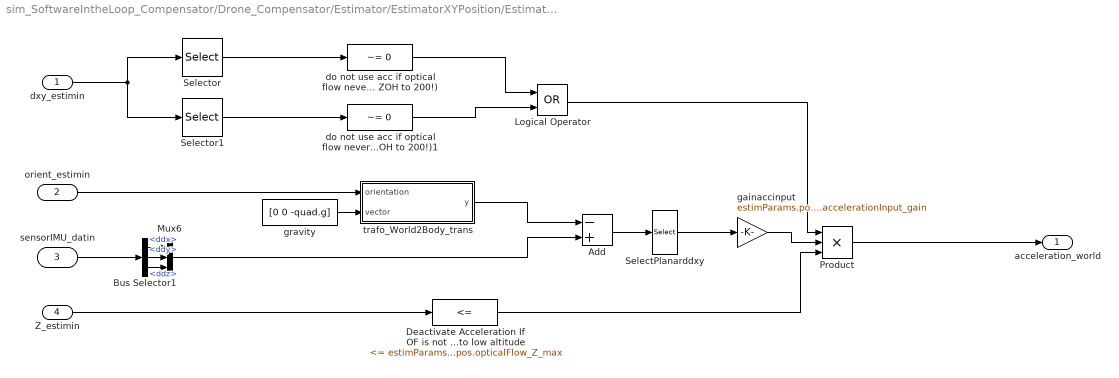
== system sim_SoftwareIntheLoop_Compensator/Drone_Compensator/Estimator/EstimatorXYPosition/EstimatorVelocity/AccelerationHandling ==
  dxy_estimin : Inport
  orient_estimin : Inport  Port=2
  sensorIMU_datin : Inport  Port=3
  Z_estimin : Inport  Port=4
  Add : Sum  Inputs=-+
  Bus Selector1 : BusSelector  OutputSignals=ddx,ddy,ddz
  Deactivate Acceleration If OF is not used due to low altitude : simulink/Logic and Bit Operations/Compare To Constant  relop=<=  const=estimParams.pos.opticalFlow_Z_max  OutDataTypeStr=boolean
  Logical Operator : Logic  Operator=OR  AllPortsSameDT=off  OutDataTypeStr=boolean
  Mux6 : Mux  Inputs=3
  Product : Product  Inputs=3
  SelectPlanarddxy : Selector  InputPortWidth=3  IndexOptions=Index vector (dialog)  Indices=[1 2]  OutputSizes=1
  Selector : Selector  InputPortWidth=2  IndexOptions=Index vector (dialog)  Indices=1  OutputSizes=1
  Selector1 : Selector  InputPortWidth=2  IndexOptions=Index vector (dialog)  Indices=2  OutputSizes=1
  do not use acc if optical flow never available (Note OF@60Hz but ZOH to 200!) : simulink/Logic and Bit Operations/Compare To Constant  relop=~=  const=0  OutDataTypeStr=boolean
  do not use acc if optical flow never available (Note OF@60Hz but ZOH to 200!)1 : simulink/Logic and Bit Operations/Compare To Constant  relop=~=  const=0  OutDataTypeStr=boolean
  gainaccinput : Gain  Gain=estimParams.pos.accelerationInput_gain
  gravity : Constant  Value=[0 0 -quad.g]
  trafo_World2Body_trans : MATLAB Function  TreatAsAtomicUnit=on
  acceleration_world : Outport
  wires:
  orient_estimin/1 -> trafo_World2Body_trans/1(orientation)
  Bus Selector1/2 -> Mux6/2  "<ddy>"
  Mux6/1 -> Add/2
  sensorIMU_datin/1 -> Bus Selector1/1
  Bus Selector1/1 -> Mux6/1  "<ddx>"
  Bus Selector1/3 -> Mux6/3  "<ddz>"
  SelectPlanarddxy/1 -> gainaccinput/1
  gainaccinput/1 -> Product/2
  gravity/1 -> trafo_World2Body_trans/2(vector)
  trafo_World2Body_trans/1(y) -> Add/1
  Add/1 -> SelectPlanarddxy/1
  Z_estimin/1 -> Deactivate Acceleration If OF is not used due to low altitude/1
  Deactivate Acceleration If OF is not used due to low altitude/1 -> Product/3
  Product/1 -> acceleration_world/1
  dxy_estimin/1 -> Selector/1, Selector1/1
  Selector/1 -> do not use acc if optical flow never available (Note OF@60Hz but ZOH to 200!)/1
  Selector1/1 -> do not use acc if optical flow never available (Note OF@60Hz but ZOH to 200!)1/1
  Logical Operator/1 -> Product/1
  do not use acc if optical flow never available (Note OF@60Hz but ZOH to 200!)/1 -> Logical Operator/1
  do not use acc if optical flow never available (Note OF@60Hz but ZOH to 200!)1/1 -> Logical Operator/2

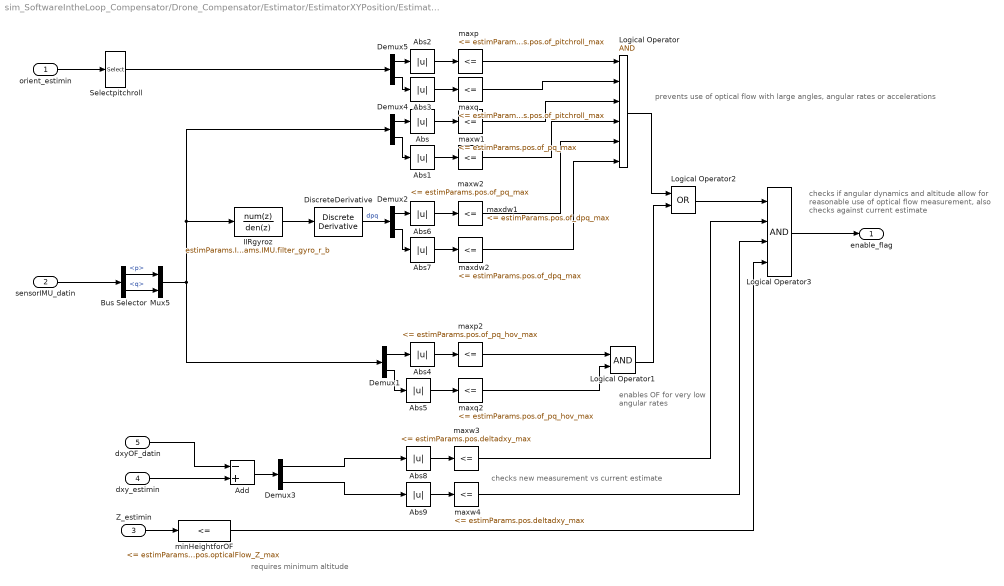
== system sim_SoftwareIntheLoop_Compensator/Drone_Compensator/Estimator/EstimatorXYPosition/EstimatorVelocity/UglyDataHandling ==
  note: requires minimum altitude
  note: checks new measurement vs current estimate
  note: checks if angular dynamics and altitude allow for
      | reasonable use of optical flow measurement,
      | also checks against current estimate
  note: enables OF for very
      | low angular rates
  note: prevents use of optical flow with large angles, angular rates or accelerations
  orient_estimin : Inport
  sensorIMU_datin : Inport  Port=2
  Z_estimin : Inport  Port=3
  dxy_estimin : Inport  Port=4
  dxyOF_datin : Inport  Port=5
  Abs{,1..9} (10 alike) : Abs
  Add : Sum  Inputs=-+
  Bus Selector : BusSelector  OutputSignals=p,q
  Demux{1..5} (5 alike) : Demux  Outputs=2
  DiscreteDerivative : simulink/Discrete/Discrete Derivative  gainval=1.0  ICPrevScaledInput=0.0  InputProcessing=Inherited  OutMin=[]  OutMax=[]  OutDataType=fixdt(1, 16)  OutScaling=2^-10  DoSatur=off
  IIRgyroz : DiscreteFilter  Numerator=estimParams.IMU.filter_gyro_r_b  Denominator=estimParams.IMU.filter_gyro_r_b
  Logical Operator : Logic  Inputs=6  AllPortsSameDT=off  OutDataTypeStr=boolean
  Logical Operator1 : Logic  AllPortsSameDT=off  OutDataTypeStr=boolean
  Logical Operator2 : Logic  Operator=OR  AllPortsSameDT=off  OutDataTypeStr=boolean
  Logical Operator3 : Logic  Inputs=4  AllPortsSameDT=off  OutDataTypeStr=boolean
  Mux5 : Mux  Inputs=2
  Selectpitchroll : Selector  InputPortWidth=3  IndexOptions=Index vector (dialog)  Indices=[2 3]  OutputSizes=1
  maxdw1 : simulink/Logic and Bit Operations/Compare To Constant  relop=<=  const=estimParams.pos.of_dpq_max  OutDataTypeStr=boolean
  maxdw2 : simulink/Logic and Bit Operations/Compare To Constant  relop=<=  const=estimParams.pos.of_dpq_max  OutDataTypeStr=boolean
  maxp : simulink/Logic and Bit Operations/Compare To Constant  relop=<=  const=estimParams.pos.of_pitchroll_max  OutDataTypeStr=boolean
  maxp2 : simulink/Logic and Bit Operations/Compare To Constant  relop=<=  const=estimParams.pos.of_pq_hov_max  OutDataTypeStr=boolean
  maxq : simulink/Logic and Bit Operations/Compare To Constant  relop=<=  const=estimParams.pos.of_pitchroll_max  OutDataTypeStr=boolean
  maxq2 : simulink/Logic and Bit Operations/Compare To Constant  relop=<=  const=estimParams.pos.of_pq_hov_max  OutDataTypeStr=boolean
  maxw1 : simulink/Logic and Bit Operations/Compare To Constant  relop=<=  const=estimParams.pos.of_pq_max  OutDataTypeStr=boolean
  maxw2 : simulink/Logic and Bit Operations/Compare To Constant  relop=<=  const=estimParams.pos.of_pq_max  OutDataTypeStr=boolean
  maxw3 : simulink/Logic and Bit Operations/Compare To Constant  relop=<=  const=estimParams.pos.deltadxy_max  OutDataTypeStr=boolean
  maxw4 : simulink/Logic and Bit Operations/Compare To Constant  relop=<=  const=estimParams.pos.deltadxy_max  OutDataTypeStr=boolean
  minHeightforOF : simulink/Logic and Bit Operations/Compare To Constant  relop=<=  const=estimParams.pos.opticalFlow_Z_max  OutDataTypeStr=boolean
  enable_flag : Outport
  wires:
  maxp2/1 -> Logical Operator1/1
  Demux5/2 -> Abs3/1
  Demux5/1 -> Abs2/1
  maxq/1 -> Logical Operator/2
  maxdw2/1 -> Logical Operator/6
  maxdw1/1 -> Logical Operator/5
  orient_estimin/1 -> Selectpitchroll/1
  maxw2/1 -> Logical Operator/4
  maxp/1 -> Logical Operator/1
  Bus Selector/2 -> Mux5/2  "<q>"
  maxq2/1 -> Logical Operator1/2
  sensorIMU_datin/1 -> Bus Selector/1
  Selectpitchroll/1 -> Demux5/1
  Bus Selector/1 -> Mux5/1  "<p>"
  maxw1/1 -> Logical Operator/3
  Logical Operator/1 -> Logical Operator2/1
  Z_estimin/1 -> minHeightforOF/1
  Abs/1 -> maxw1/1
  Abs1/1 -> maxw2/1
  Demux4/1 -> Abs/1
  Demux4/2 -> Abs1/1
  Abs2/1 -> maxp/1
  Abs3/1 -> maxq/1
  Abs4/1 -> maxp2/1
  Abs5/1 -> maxq2/1
  Demux1/1 -> Abs4/1
  Demux1/2 -> Abs5/1
  Logical Operator1/1 -> Logical Operator2/2
  Abs6/1 -> maxdw1/1
  Abs7/1 -> maxdw2/1
  Demux2/1 -> Abs6/1
  Demux2/2 -> Abs7/1
  DiscreteDerivative/1 -> Demux2/1  "dpq"
  Logical Operator3/1 -> enable_flag/1
  Logical Operator2/1 -> Logical Operator3/1
  Abs8/1 -> maxw3/1
  Abs9/1 -> maxw4/1
  Add/1 -> Demux3/1
  dxy_estimin/1 -> Add/2
  Demux3/1 -> Abs8/1
  Demux3/2 -> Abs9/1
  dxyOF_datin/1 -> Add/1
  maxw3/1 -> Logical Operator3/2
  maxw4/1 -> Logical Operator3/3
  Mux5/1 -> Demux4/1, IIRgyroz/1, Demux1/1
  IIRgyroz/1 -> DiscreteDerivative/1
  minHeightforOF/1 -> Logical Operator3/4

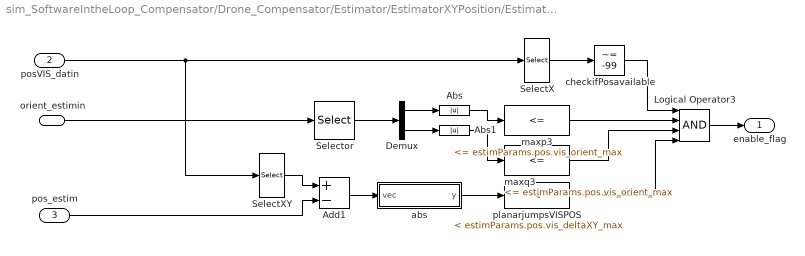
== system sim_SoftwareIntheLoop_Compensator/Drone_Compensator/Estimator/EstimatorXYPosition/EstimatorXYPosition/OutlierHandling ==
  orient_estimin : Inport
  posVIS_datin : Inport  Port=2
  pos_estim : Inport  Port=3
  Abs : Abs
  Abs1 : Abs
  Add1 : Sum  Inputs=+-
  Demux : Demux  Outputs=2
  Logical Operator3 : Logic  Inputs=4  AllPortsSameDT=off  OutDataTypeStr=boolean
  SelectX : Selector  InputPortWidth=4  IndexOptions=Index vector (dialog)  Indices=[1]  OutputSizes=1
  SelectXY : Selector  InputPortWidth=4  IndexOptions=Index vector (dialog)  Indices=[1 2]  OutputSizes=1
  Selector : Selector  InputPortWidth=3  IndexOptions=Index vector (dialog)  Indices=[2 3]  OutputSizes=1
  abs : MATLAB Function  TreatAsAtomicUnit=on
  checkifPosavailable : simulink/Logic and Bit Operations/Compare To Constant  relop=~=  const=-99  OutDataTypeStr=boolean
  maxp3 : simulink/Logic and Bit Operations/Compare To Constant  relop=<=  const=estimParams.pos.vis_orient_max  OutDataTypeStr=boolean
  maxq3 : simulink/Logic and Bit Operations/Compare To Constant  relop=<=  const=estimParams.pos.vis_orient_max  OutDataTypeStr=boolean
  planarjumpsVISPOS : simulink/Logic and Bit Operations/Compare To Constant  relop=<  const=estimParams.pos.vis_deltaXY_max  OutDataTypeStr=boolean
  enable_flag : Outport
  wires:
  posVIS_datin/1 -> SelectXY/1, SelectX/1
  SelectX/1 -> checkifPosavailable/1
  checkifPosavailable/1 -> Logical Operator3/1
  Logical Operator3/1 -> enable_flag/1
  maxp3/1 -> Logical Operator3/2
  maxq3/1 -> Logical Operator3/3
  SelectXY/1 -> Add1/1
  Add1/1 -> abs/1(vec)
  pos_estim/1 -> Add1/2
  abs/1(y) -> planarjumpsVISPOS/1
  planarjumpsVISPOS/1 -> Logical Operator3/4
  orient_estimin/1 -> Selector/1
  Selector/1 -> Demux/1
  Demux/1 -> Abs/1
  Demux/2 -> Abs1/1
  Abs/1 -> maxp3/1
  Abs1/1 -> maxq3/1

== matlab function sim_SoftwareIntheLoop_Compensator/Drone_Compensator/ControllerLQR/FullstateController/MATLAB Function ==
  data: K input; x input; u output
function u = fcn(K,x)
u= -K*x;
